simulink model "sampleModel152"  (Simulink 9.1)
settings: Solver=VariableStepAuto  StartTime=0.0  StopTime=10.0  RelTol=1e-3
undefined symbols (not defined in the file): DiscIntNeverNeededParam, Newton, Raphson
libraries: simulink x17
settings Model: Creator=DELL  LastModifiedBy=DELL
settings DataIOCC: SaveFormat=Dataset
settings OptimizationCC: LifeSpan=auto
settings DebuggingCC: UnderspecifiedInitializationDetection=Simplified  MergeDetectMultiDrivingBlocksExec=error  SFUnexpectedBacktrackingDiag=error  SFNoUnconditionalDefaultTransitionDiag=error  SFExecutionAtInitializationDiag=warning
settings HardwareCC: ProdBitPerPointer=64  ProdBitPerSizeT=64  ProdBitPerPtrDiffT=64  ProdLargestAtomicFloat=Float  ProdIntDivRoundTo=Zero  ProdEndianess=LittleEndian  ProdWordSize=64  ProdHWDeviceType=Intel->x86-64 (Windows64)
settings ModelReferenceCC: PropagateSignalLabelsOutOfModel=on
settings CodeAppCC: StateflowObjectComments=off
settings GRTTargetCC: TargetLangStandard=C99 (ISO)  CombineOutputUpdateFcns=on  GRTInterface=off
settings ConfigComp: CovMetricSettings=dwe  CovHtmlReporting=off  CovSaveCumulativeToWorkspaceVar=off  CovSaveSingleToWorkspaceVar=off  CovExternalEMLEnable=on

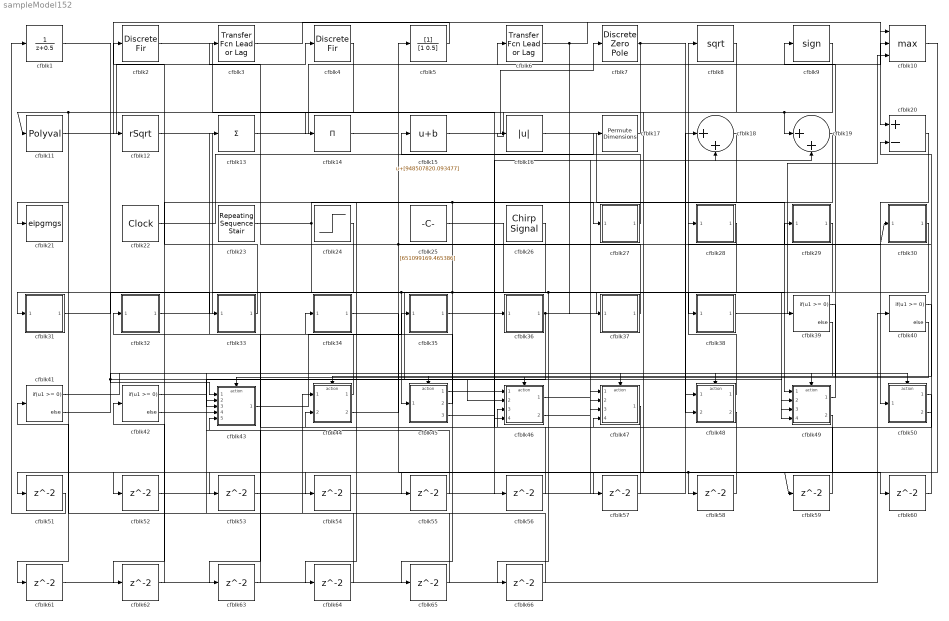
== system sampleModel152 ==
  cfblk1 : DiscreteTransferFcn  SampleTime=1
  cfblk10 : MinMax  Function=max  Inputs=3
  cfblk11 : Polyval  Coefs=[ +2.081618890e-019, -1.441693666e-014, +4.719686976e-010, -8.536869453e-006, +1.621573104e-001, -8.087801117e+001 ]
  cfblk12 : Sqrt  Operator=rSqrt  AlgorithmType=Newton-Raphson  SaturateOnIntegerOverflow=on
  cfblk13 : Sum  Inputs=+
  cfblk14 : Product  Inputs=*
  cfblk15 : Bias  Bias=[948507820.093477]
  cfblk16 : Abs
  cfblk17 : PermuteDimensions
  cfblk18 : Sum  Inputs=|++
  cfblk19 : Sum  Inputs=|++
  cfblk2 : DiscreteFir  SampleTime=1
  cfblk20 : Sum  Inputs=+-
  cfblk21 : ToWorkspace  VariableName=eipgmgs  SaveFormat=Timeseries  SampleTime=-1
  cfblk22 : DigitalClock
  cfblk23 : simulink/Sources/Repeating Sequence Stair  OutValues=[-106869927.062415, -61159748.069920]  tsamp=-1  OutMin=[]  OutMax=[]  OutDataTypeStr=double  OutputDataTypeScalingMode=double  OutDataType=fixdt(0,8)  ConRadixGroup=Best Precision: Vector-wise  OutScaling=2^-12
  cfblk24 : Step  Time=[15.000000]  Before=[-172570946.840389]  After=[-976275544.240260]  SampleTime=0
  cfblk25 : Constant  Value=[651099169.465386]  SampleTime=1
  cfblk26 : simulink/Sources/Chirp Signal  f1=[-435057966.777252]  T=[115531586.665615]  f2=[491750431.839140]
  cfblk27 : Subsystem
  cfblk28 : Subsystem
  cfblk29 : Subsystem
  cfblk3 : simulink/Discrete/Transfer Fcn Lead or Lag  PoleZ=0.95  ZeroZ=0.75  ICPrevOutput=0.0  ICPrevInput=0.0  DoSatur=off
      settings: SourceProductName=Simulink  SourceProductBaseCode=SL
  cfblk30 : Subsystem
  cfblk31 : Subsystem
  cfblk32 : Subsystem
  cfblk33 : Subsystem
  cfblk34 : Subsystem
  cfblk35 : Subsystem
  cfblk36 : Subsystem
  cfblk37 : Subsystem
  cfblk38 : Subsystem
  cfblk{39..42} (4 alike) : If  IfExpression=u1 >= 0  SampleTime=1
  cfblk4 : DiscreteFir  SampleTime=1
  cfblk43 : Subsystem  TreatAsAtomicUnit=on
  cfblk44 : Subsystem  TreatAsAtomicUnit=on
  cfblk45 : Subsystem  TreatAsAtomicUnit=on
  cfblk46 : Subsystem  TreatAsAtomicUnit=on
  cfblk47 : Subsystem  TreatAsAtomicUnit=on
  cfblk48 : Subsystem  TreatAsAtomicUnit=on
  cfblk49 : Subsystem  TreatAsAtomicUnit=on
  cfblk5 : DiscreteFilter  SampleTime=1
  cfblk50 : Subsystem  TreatAsAtomicUnit=on
  cfblk{51..66} (16 alike) : Delay  SampleTime=1
  cfblk6 : simulink/Discrete/Transfer Fcn Lead or Lag  PoleZ=0.95  ZeroZ=0.75  ICPrevOutput=0.0  ICPrevInput=0.0  DoSatur=off
      settings: SourceProductName=Simulink  SourceProductBaseCode=SL
  cfblk7 : DiscreteZeroPole  Poles=[0 0.5]  Gain=1
  cfblk8 : Sqrt  SaturateOnIntegerOverflow=on
  cfblk9 : Signum
  wires:
  cfblk13/1 -> cfblk6/1
  cfblk50/1(cfblk2) -> cfblk32/1(cfblk1)
  cfblk11/1 -> cfblk4/1
  cfblk27/1(cfblk2) -> cfblk15/1
  cfblk12/1 -> cfblk46/2(cfblk14)
  cfblk15/1 -> cfblk7/1
  cfblk6/1 -> cfblk20/1, cfblk37/1(cfblk1)
  cfblk5/1 -> cfblk12/1
  cfblk17/1 -> cfblk16/1
  cfblk33/1(cfblk2) -> cfblk2/1
  cfblk23/1 -> cfblk27/1(cfblk1), cfblk49/4(cfblk16)
  cfblk9/1 -> cfblk19/1, cfblk57/1
  cfblk1/1 -> cfblk48/2(cfblk8), cfblk43/1(cfblk1)
  cfblk8/1 -> cfblk11/1, cfblk21/1
  cfblk44/1(cfblk2) -> cfblk13/1
  cfblk22/1 -> cfblk5/1
  cfblk45/1(cfblk2) -> cfblk19/2
  cfblk48/1(cfblk2) -> cfblk8/1
  cfblk2/1 -> cfblk36/1(cfblk1)
  cfblk28/1(cfblk2) -> cfblk45/1(cfblk1), cfblk63/1
  cfblk43/1(cfblk2) -> cfblk35/1(cfblk1)
  cfblk3/1 -> cfblk10/1
  cfblk50/2(cfblk17) -> cfblk28/1(cfblk1)
  cfblk19/1 -> cfblk54/1, cfblk55/1
  cfblk16/1 -> cfblk49/1(cfblk1)
  cfblk14/1 -> cfblk10/2
  cfblk24/1 -> cfblk31/1(cfblk1)
  cfblk32/1(cfblk2) -> cfblk38/1(cfblk1)
  cfblk49/1(cfblk2) -> cfblk9/1
  cfblk7/1 -> cfblk49/2(cfblk14), cfblk14/1
  cfblk44/2(cfblk7) -> cfblk17/1, cfblk30/1(cfblk1)
  cfblk38/1(cfblk2) -> cfblk10/3
  cfblk31/1(cfblk2) -> cfblk33/1(cfblk1)
  cfblk36/1(cfblk2) -> cfblk39/1, cfblk43/3(cfblk11)
  cfblk20/1 -> cfblk50/1(cfblk1)
  cfblk30/1(cfblk2) -> cfblk64/1, cfblk65/1, cfblk66/1
  cfblk45/2(cfblk11) -> cfblk34/1(cfblk1)
  cfblk47/1(cfblk2) -> cfblk46/3(cfblk15)
  cfblk48/2(cfblk9) -> cfblk44/2(cfblk6)
  cfblk26/1 -> cfblk46/4(cfblk16)
  cfblk34/1(cfblk2) -> cfblk58/1, cfblk59/1
  cfblk46/1(cfblk2) -> cfblk29/1(cfblk1)
  cfblk37/1(cfblk2) -> cfblk3/1
  cfblk25/1 -> cfblk49/3(cfblk15)
  cfblk46/2(cfblk17) -> cfblk18/2
  cfblk39/1 -> cfblk43/Action
  cfblk39/2 -> cfblk44/Action
  cfblk40/1 -> cfblk45/Action
  cfblk40/2 -> cfblk46/Action
  cfblk41/1 -> cfblk47/Action
  cfblk41/2 -> cfblk48/Action
  cfblk42/1 -> cfblk49/Action
  cfblk42/2 -> cfblk50/Action
  cfblk4/1 -> cfblk51/1
  cfblk51/1 -> cfblk1/1
  cfblk10/1 -> cfblk52/1
  cfblk52/1 -> cfblk47/1(cfblk1)
  cfblk29/1(cfblk2) -> cfblk53/1
  cfblk53/1 -> cfblk48/1(cfblk1)
  cfblk54/1 -> cfblk18/1
  cfblk55/1 -> cfblk43/2(cfblk10)
  cfblk35/1(cfblk2) -> cfblk56/1
  cfblk56/1 -> cfblk46/1(cfblk1)
  cfblk57/1 -> cfblk47/3(cfblk14)
  cfblk58/1 -> cfblk47/2(cfblk13)
  cfblk59/1 -> cfblk47/4(cfblk15)
  cfblk45/3(cfblk12) -> cfblk60/1
  cfblk60/1 -> cfblk20/2
  cfblk49/2(cfblk17) -> cfblk61/1
  cfblk61/1 -> cfblk40/1
  cfblk18/1 -> cfblk62/1
  cfblk62/1 -> cfblk42/1
  cfblk63/1 -> cfblk43/5(cfblk13)
  cfblk64/1 -> cfblk44/1(cfblk1)
  cfblk65/1 -> cfblk41/1
  cfblk66/1 -> cfblk43/4(cfblk12)

== system sampleModel152/cfblk27 ==
  cfblk1 : Inport
  cfblk2 : Outport
  wires:
  cfblk1/1 -> cfblk2/1

== system sampleModel152/cfblk28 ==
  cfblk1 : Inport
  cfblk2 : Outport
  wires:
  cfblk1/1 -> cfblk2/1

== system sampleModel152/cfblk29 ==
  cfblk1 : Inport
  cfblk2 : Outport
  wires:
  cfblk1/1 -> cfblk2/1

== system sampleModel152/cfblk30 ==
  cfblk1 : Inport
  cfblk2 : Outport
  wires:
  cfblk1/1 -> cfblk2/1

== system sampleModel152/cfblk31 ==
  cfblk1 : Inport
  cfblk2 : Outport
  wires:
  cfblk1/1 -> cfblk2/1

== system sampleModel152/cfblk32 ==
  cfblk1 : Inport
  cfblk2 : Outport
  wires:
  cfblk1/1 -> cfblk2/1

== system sampleModel152/cfblk33 ==
  cfblk1 : Inport
  cfblk2 : Outport
  wires:
  cfblk1/1 -> cfblk2/1

== system sampleModel152/cfblk34 ==
  cfblk1 : Inport
  cfblk2 : Outport
  wires:
  cfblk1/1 -> cfblk2/1

== system sampleModel152/cfblk35 ==
  cfblk1 : Inport
  cfblk2 : Outport
  wires:
  cfblk1/1 -> cfblk2/1

== system sampleModel152/cfblk36 ==
  cfblk1 : Inport
  cfblk2 : Outport
  wires:
  cfblk1/1 -> cfblk2/1

== system sampleModel152/cfblk37 ==
  cfblk1 : Inport
  cfblk2 : Outport
  wires:
  cfblk1/1 -> cfblk2/1

== system sampleModel152/cfblk38 ==
  cfblk1 : Inport
  cfblk2 : Outport
  wires:
  cfblk1/1 -> cfblk2/1

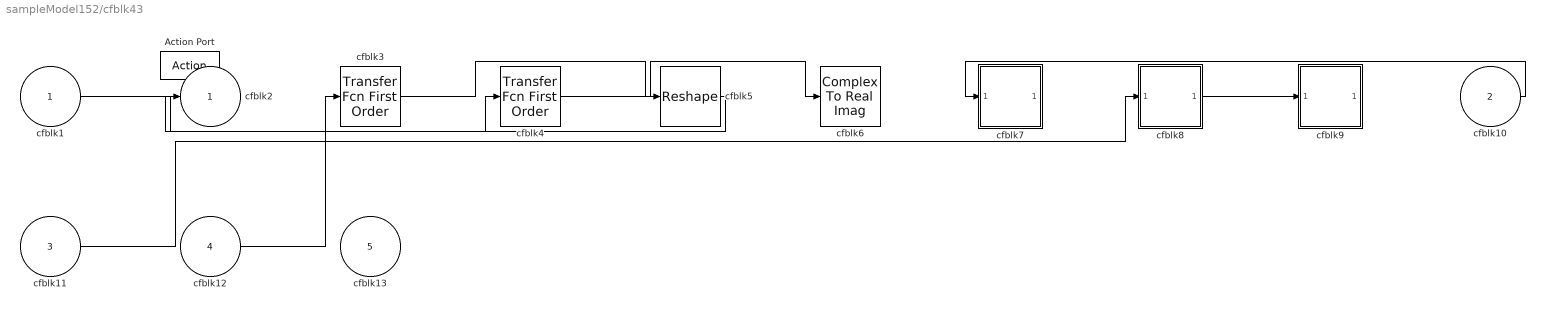
== system sampleModel152/cfblk43 ==
  cfblk1 : Inport
  cfblk10 : Inport  Port=2
  cfblk11 : Inport  Port=3
  cfblk12 : Inport  Port=4
  cfblk13 : Inport  Port=5
  Action Port : ActionPort  ActionType=then
  cfblk3 : simulink/Discrete/Transfer Fcn First Order  PoleZ=0.95  ICPrevOutput=0.0  DoSatur=off
      settings: SourceProductName=Simulink
  cfblk4 : simulink/Discrete/Transfer Fcn First Order  PoleZ=0.95  ICPrevOutput=0.0  DoSatur=off
      settings: SourceProductName=Simulink
  cfblk5 : Reshape
  cfblk6 : ComplexToRealImag
  cfblk7 : Subsystem
  cfblk8 : Subsystem
  cfblk9 : Subsystem
  cfblk2 : Outport
  wires:
  cfblk1/1 -> cfblk4/1
  cfblk11/1 -> cfblk8/1(cfblk1)
  cfblk4/1 -> cfblk6/1
  cfblk10/1 -> cfblk7/1(cfblk1)
  cfblk8/1(cfblk2) -> cfblk9/1(cfblk1)
  cfblk3/1 -> cfblk5/1
  cfblk12/1 -> cfblk3/1
  cfblk5/1 -> cfblk2/1

== system sampleModel152/cfblk44 ==
  cfblk1 : Inport
  cfblk6 : Inport  Port=2
  Action Port : ActionPort  ActionType=else
  cfblk3 : simulink/Continuous/PID Controller  Controller=PID  TimeDomain=Discrete-time  SampleTime=-1  IntegratorMethod=Forward Euler  FilterMethod=Forward Euler  Form=Parallel  UseFilter=on  ControllerParametersSource=internal  P=1  I=1  D=0  N=100  InitialConditionSource=internal  InitialConditionForIntegrator=0  InitialConditionForFilter=0  ExternalReset=none  LimitOutput=off  UpperSaturationLimit=inf  LowerSaturationLimit=-inf  LinearizeAsGain=off  AntiWindupMode=none  Kb=1  TrackingMode=off  Kt=1  PParamMin=[]  PParamMax=[]  IParamMin=[]  IParamMax=[]  DParamMin=[]  DParamMax=[]  NParamMin=[]  NParamMax=[]  KbParamMin=[]  KbParamMax=[]  KtParamMin=[]  KtParamMax=[]  POutMin=[]  POutMax=[]  IOutMin=[]  IOutMax=[]  DOutMin=[]  DOutMax=[]  NOutMin=[]  NOutMax=[]  KbOutMin=[]  KbOutMax=[]  KtOutMin=[]  KtOutMax=[]  IntegratorOutMin=[]  IntegratorOutMax=[]  FilterOutMin=[]  FilterOutMax=[]  SumOutMin=[]  SumOutMax=[]  SumI1OutMin=[]  SumI1OutMax=[]  SumI2OutMin=[]  SumI2OutMax=[]  SumI3OutMin=[]  SumI3OutMax=[]  SumDOutMin=[]  SumDOutMax=[]  SaturationOutMin=[]  SaturationOutMax=[]  IntegratorContinuousStateAttributes=''  IntegratorStateMustResolveToSignalObject=off  IntegratorRTWStateStorageClass=Auto  FilterContinuousStateAttributes=''  FilterStateMustResolveToSignalObject=off  FilterRTWStateStorageClass=Auto  DifferentiatorICPrevScaledInput=0  DifferentiatorOutMin=[]  DifferentiatorOutMax=[]  FilterDiffOutCoefMin=[]  FilterDiffOutCoefMax=[]  SumDenOutMin=[]  SumDenOutMax=[]  SumNumOutMin=[]  SumNumOutMax=[]  ReciprocalOutMin=[]  ReciprocalOutMax=[]  DivideOutMin=[]  DivideOutMax=[]  TunerSelectOption=Transfer Function Based (PID Tuner App)
  cfblk4 : DiscreteZeroPole  Poles=[0 0.5]  Gain=1  SampleTime=-1
  cfblk5 : simulink/Math Operations/Slider Gain  gain=1  low=0  high=2
  cfblk2 : Outport
  cfblk7 : Outport  Port=2
  wires:
  cfblk6/1 -> cfblk2/1
  cfblk5/1 -> cfblk7/1
  cfblk4/1 -> cfblk3/1
  cfblk1/1 -> cfblk4/1
  cfblk3/1 -> cfblk5/1

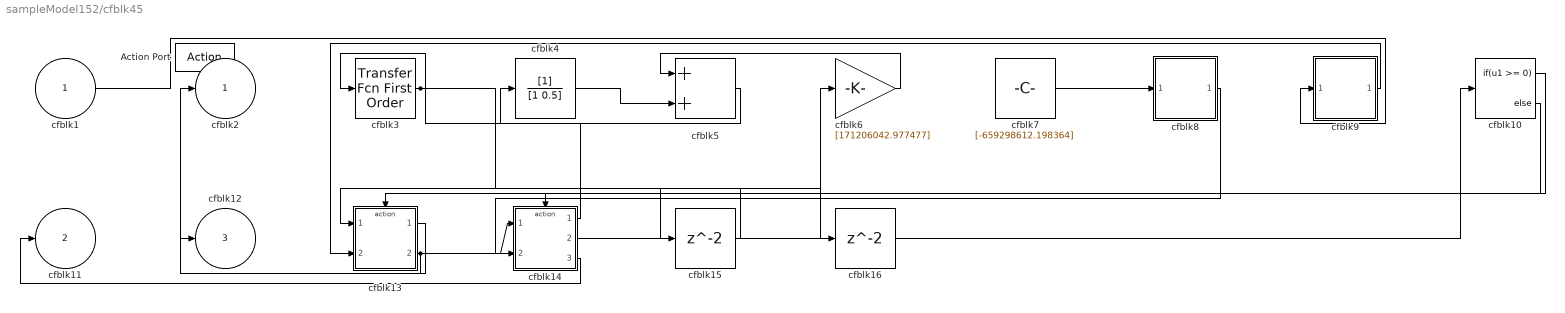
== system sampleModel152/cfblk45 ==
  cfblk1 : Inport
  Action Port : ActionPort  ActionType=then
  cfblk10 : If  IfExpression=u1 >= 0  SampleTime=1
  cfblk13 : Subsystem  TreatAsAtomicUnit=on
  cfblk14 : Subsystem  TreatAsAtomicUnit=on
  cfblk15 : Delay
  cfblk16 : Delay
  cfblk3 : simulink/Discrete/Transfer Fcn First Order  PoleZ=0.95  ICPrevOutput=0.0  DoSatur=off
      settings: SourceProductName=Simulink
  cfblk4 : DiscreteFilter
  cfblk5 : Sum
  cfblk6 : Gain  Gain=[171206042.977477]
  cfblk7 : Constant  Value=[-659298612.198364]  SampleTime=1
  cfblk8 : Subsystem
  cfblk9 : Subsystem
  cfblk2 : Outport
  cfblk11 : Outport  Port=2
  cfblk12 : Outport  Port=3
  wires:
  cfblk3/1 -> cfblk15/1, cfblk16/1
  cfblk6/1 -> cfblk5/1
  cfblk13/1(cfblk2) -> cfblk2/1
  cfblk5/1 -> cfblk3/1
  cfblk14/1(cfblk2) -> cfblk4/1
  cfblk14/2(cfblk8) -> cfblk6/1
  cfblk13/2(cfblk10) -> cfblk14/1(cfblk1), cfblk12/1
  cfblk9/1(cfblk2) -> cfblk13/2(cfblk9)
  cfblk1/1 -> cfblk9/1(cfblk1)
  cfblk14/3(cfblk9) -> cfblk11/1
  cfblk4/1 -> cfblk5/2
  cfblk8/1(cfblk2) -> cfblk14/2(cfblk7)
  cfblk7/1 -> cfblk8/1(cfblk1)
  cfblk10/1 -> cfblk13/Action
  cfblk10/2 -> cfblk14/Action
  cfblk15/1 -> cfblk13/1(cfblk1)
  cfblk16/1 -> cfblk10/1

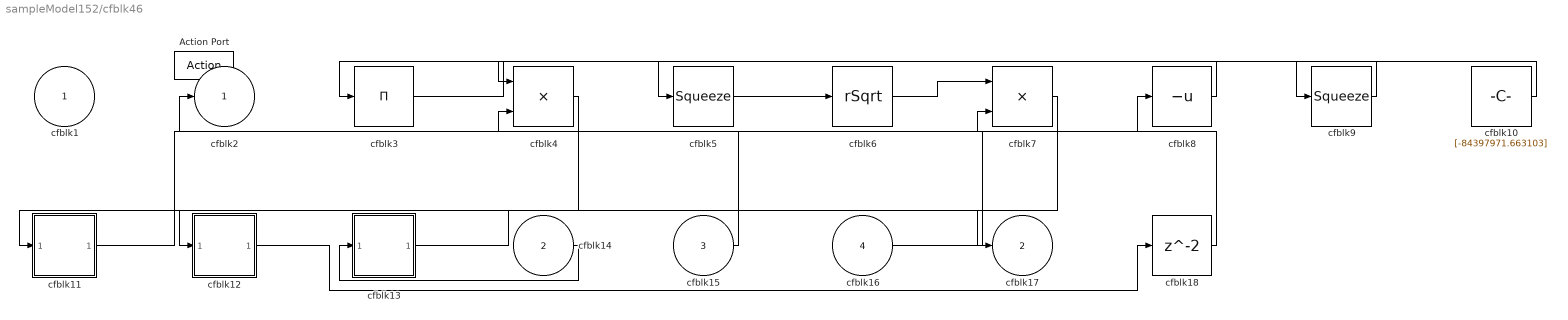
== system sampleModel152/cfblk46 ==
  cfblk1 : Inport
  cfblk14 : Inport  Port=2
  cfblk15 : Inport  Port=3
  cfblk16 : Inport  Port=4
  Action Port : ActionPort  ActionType=else
  cfblk10 : Constant  Value=[-84397971.663103]  SampleTime=1
  cfblk11 : Subsystem
  cfblk12 : Subsystem
  cfblk13 : Subsystem
  cfblk18 : Delay
  cfblk3 : Product  Inputs=*
  cfblk4 : Product
  cfblk5 : Squeeze
  cfblk6 : Sqrt  Operator=rSqrt  AlgorithmType=Newton-Raphson  SaturateOnIntegerOverflow=on
  cfblk7 : Product  Inputs=**
  cfblk8 : UnaryMinus
  cfblk9 : Squeeze
  cfblk2 : Outport
  cfblk17 : Outport  Port=2
  wires:
  cfblk4/1 -> cfblk11/1(cfblk1)
  cfblk14/1 -> cfblk13/1(cfblk1)
  cfblk16/1 -> cfblk8/1
  cfblk13/1(cfblk2) -> cfblk17/1
  cfblk15/1 -> cfblk2/1
  cfblk5/1 -> cfblk6/1
  cfblk10/1 -> cfblk5/1
  cfblk8/1 -> cfblk3/1
  cfblk7/1 -> cfblk12/1(cfblk1)
  cfblk6/1 -> cfblk7/1
  cfblk11/1(cfblk2) -> cfblk7/2
  cfblk3/1 -> cfblk9/1
  cfblk9/1 -> cfblk4/1
  cfblk12/1(cfblk2) -> cfblk18/1
  cfblk18/1 -> cfblk4/2

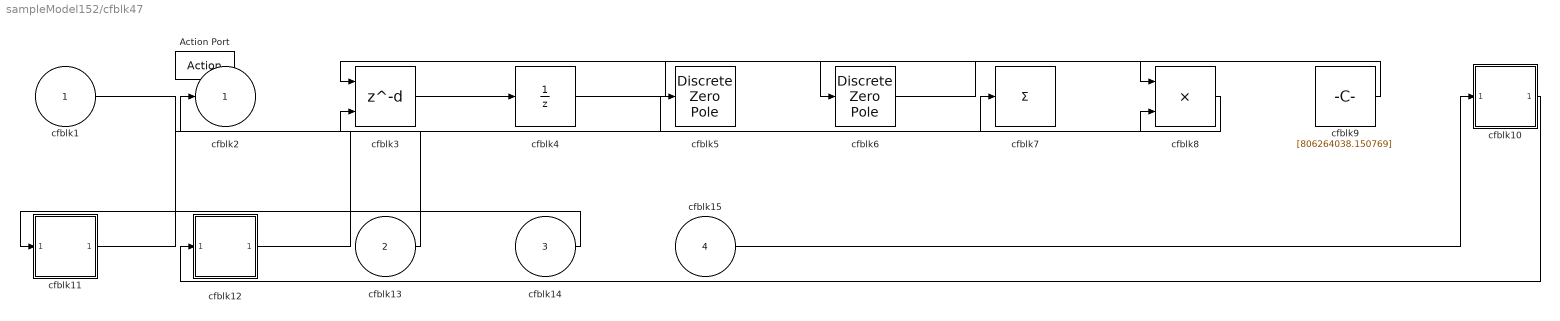
== system sampleModel152/cfblk47 ==
  cfblk1 : Inport
  cfblk13 : Inport  Port=2
  cfblk14 : Inport  Port=3
  cfblk15 : Inport  Port=4
  Action Port : ActionPort  ActionType=then
  cfblk10 : Subsystem
  cfblk11 : Subsystem
  cfblk12 : Subsystem
  cfblk3 : Delay  DelayLengthSource=Input port
      settings: InputPortMap=u0,p1
  cfblk4 : UnitDelay  SampleTime=-1
  cfblk5 : DiscreteZeroPole  Poles=[0 0.5]  Gain=1  SampleTime=-1
  cfblk6 : DiscreteZeroPole  Poles=[0 0.5]  Gain=1  SampleTime=-1
  cfblk7 : Sum  Inputs=+
  cfblk8 : Product
  cfblk9 : Constant  Value=[806264038.150769]  SampleTime=1
  cfblk2 : Outport
  wires:
  cfblk12/1(cfblk2) -> cfblk7/1
  cfblk9/1 -> cfblk3/1
  cfblk15/1 -> cfblk10/1(cfblk1)
  cfblk10/1(cfblk2) -> cfblk12/1(cfblk1)
  cfblk6/1 -> cfblk8/1
  cfblk3/1 -> cfblk4/1
  cfblk11/1(cfblk2) -> cfblk8/2
  cfblk8/1 -> cfblk2/1
  cfblk14/1 -> cfblk11/1(cfblk1)
  cfblk4/1 -> cfblk6/1
  cfblk1/1 -> cfblk5/1
  cfblk13/1 -> cfblk3/2

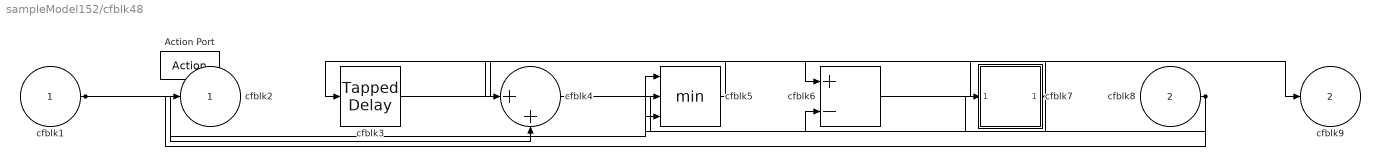
== system sampleModel152/cfblk48 ==
  cfblk1 : Inport
  cfblk8 : Inport  Port=2
  Action Port : ActionPort  ActionType=else
  cfblk3 : simulink/Discrete/Tapped Delay  vinit=0.0  samptime=-1  NumDelays=1  DelayOrder=Oldest  includeCurrent=off
  cfblk4 : Sum  Inputs=|++
  cfblk5 : MinMax  Inputs=3
  cfblk6 : Sum  Inputs=+-
  cfblk7 : Subsystem
  cfblk2 : Outport
  cfblk9 : Outport  Port=2
  wires:
  cfblk6/1 -> cfblk9/1
  cfblk5/1 -> cfblk3/1
  cfblk8/1 -> cfblk7/1(cfblk1), cfblk5/3, cfblk2/1
  cfblk1/1 -> cfblk5/1, cfblk4/2
  cfblk3/1 -> cfblk6/1
  cfblk7/1(cfblk2) -> cfblk4/1, cfblk5/2
  cfblk4/1 -> cfblk6/2

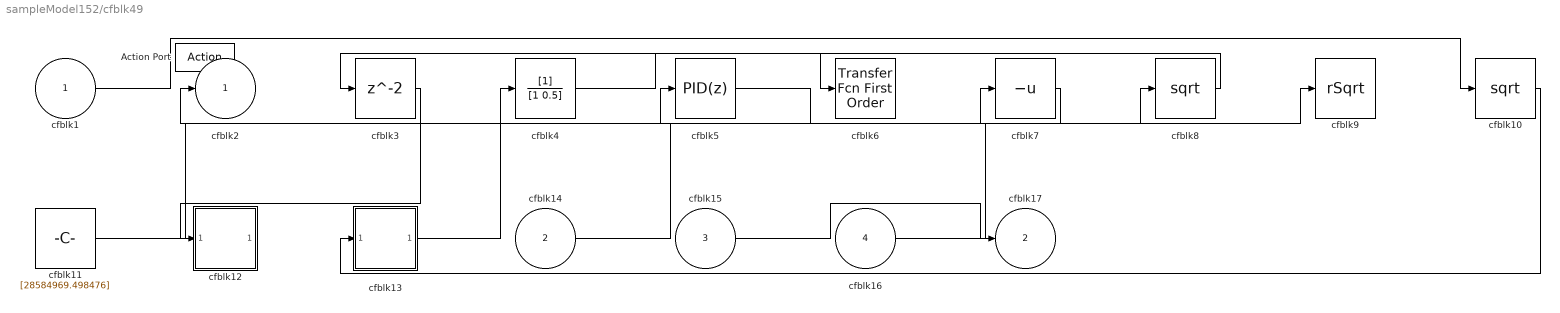
== system sampleModel152/cfblk49 ==
  cfblk1 : Inport
  cfblk14 : Inport  Port=2
  cfblk15 : Inport  Port=3
  cfblk16 : Inport  Port=4
  Action Port : ActionPort  ActionType=then
  cfblk10 : Sqrt  SaturateOnIntegerOverflow=on
  cfblk11 : Constant  Value=[28584969.498476]  SampleTime=1
  cfblk12 : Subsystem
  cfblk13 : Subsystem
  cfblk3 : Delay
  cfblk4 : DiscreteFilter
  cfblk5 : simulink/Continuous/PID Controller  Controller=PID  TimeDomain=Discrete-time  SampleTime=-1  IntegratorMethod=Forward Euler  FilterMethod=Forward Euler  Form=Parallel  UseFilter=on  ControllerParametersSource=internal  P=1  I=1  D=0  N=100  InitialConditionSource=internal  InitialConditionForIntegrator=0  InitialConditionForFilter=0  ExternalReset=none  LimitOutput=off  UpperSaturationLimit=inf  LowerSaturationLimit=-inf  LinearizeAsGain=off  AntiWindupMode=none  Kb=1  TrackingMode=off  Kt=1  PParamMin=[]  PParamMax=[]  IParamMin=[]  IParamMax=[]  DParamMin=[]  DParamMax=[]  NParamMin=[]  NParamMax=[]  KbParamMin=[]  KbParamMax=[]  KtParamMin=[]  KtParamMax=[]  POutMin=[]  POutMax=[]  IOutMin=[]  IOutMax=[]  DOutMin=[]  DOutMax=[]  NOutMin=[]  NOutMax=[]  KbOutMin=[]  KbOutMax=[]  KtOutMin=[]  KtOutMax=[]  IntegratorOutMin=[]  IntegratorOutMax=[]  FilterOutMin=[]  FilterOutMax=[]  SumOutMin=[]  SumOutMax=[]  SumI1OutMin=[]  SumI1OutMax=[]  SumI2OutMin=[]  SumI2OutMax=[]  SumI3OutMin=[]  SumI3OutMax=[]  SumDOutMin=[]  SumDOutMax=[]  SaturationOutMin=[]  SaturationOutMax=[]  IntegratorContinuousStateAttributes=''  IntegratorStateMustResolveToSignalObject=off  IntegratorRTWStateStorageClass=Auto  FilterContinuousStateAttributes=''  FilterStateMustResolveToSignalObject=off  FilterRTWStateStorageClass=Auto  DifferentiatorICPrevScaledInput=0  DifferentiatorOutMin=[]  DifferentiatorOutMax=[]  FilterDiffOutCoefMin=[]  FilterDiffOutCoefMax=[]  SumDenOutMin=[]  SumDenOutMax=[]  SumNumOutMin=[]  SumNumOutMax=[]  ReciprocalOutMin=[]  ReciprocalOutMax=[]  DivideOutMin=[]  DivideOutMax=[]  TunerSelectOption=Transfer Function Based (PID Tuner App)
  cfblk6 : simulink/Discrete/Transfer Fcn First Order  PoleZ=0.95  ICPrevOutput=0.0  DoSatur=off
      settings: SourceProductName=Simulink
  cfblk7 : UnaryMinus
  cfblk8 : Sqrt  SaturateOnIntegerOverflow=on
  cfblk9 : Sqrt  Operator=rSqrt  AlgorithmType=Newton-Raphson  SaturateOnIntegerOverflow=on
  cfblk2 : Outport
  cfblk17 : Outport  Port=2
  wires:
  cfblk8/1 -> cfblk3/1
  cfblk11/1 -> cfblk5/1
  cfblk4/1 -> cfblk6/1
  cfblk5/1 -> cfblk9/1
  cfblk1/1 -> cfblk10/1
  cfblk16/1 -> cfblk8/1
  cfblk10/1 -> cfblk13/1(cfblk1)
  cfblk7/1 -> cfblk2/1
  cfblk13/1(cfblk2) -> cfblk4/1
  cfblk3/1 -> cfblk12/1(cfblk1)
  cfblk14/1 -> cfblk7/1
  cfblk15/1 -> cfblk17/1

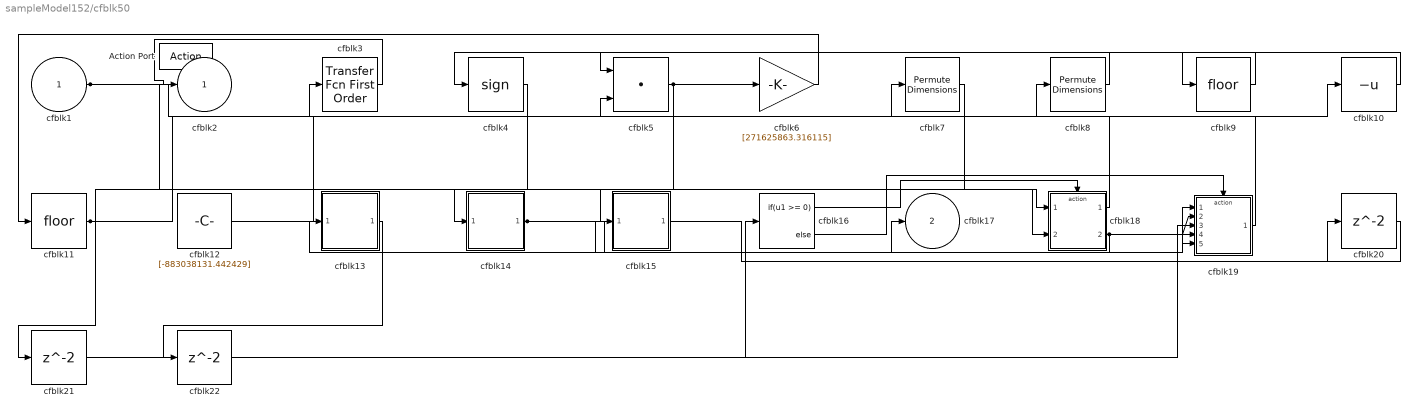
== system sampleModel152/cfblk50 ==
  cfblk1 : Inport
  Action Port : ActionPort  ActionType=else
  cfblk10 : UnaryMinus
  cfblk11 : Rounding
  cfblk12 : Constant  Value=[-883038131.442429]  SampleTime=1
  cfblk13 : Subsystem
  cfblk14 : Subsystem
  cfblk15 : Subsystem
  cfblk16 : If  IfExpression=u1 >= 0  SampleTime=1
  cfblk18 : Subsystem  TreatAsAtomicUnit=on
  cfblk19 : Subsystem  TreatAsAtomicUnit=on
  cfblk20 : Delay
  cfblk21 : Delay
  cfblk22 : Delay
  cfblk3 : simulink/Discrete/Transfer Fcn First Order  PoleZ=0.95  ICPrevOutput=0.0  DoSatur=off
      settings: SourceProductName=Simulink
  cfblk4 : Signum
  cfblk5 : DotProduct  InputSameDT=on  OutDataTypeStr=Inherit: Inherit via internal rule
  cfblk6 : Gain  Gain=[271625863.316115]
  cfblk7 : PermuteDimensions
  cfblk8 : PermuteDimensions
  cfblk9 : Rounding
  cfblk2 : Outport
  cfblk17 : Outport  Port=2
  wires:
  cfblk1/1 -> cfblk10/1, cfblk18/2(cfblk11)
  cfblk3/1 -> cfblk2/1
  cfblk6/1 -> cfblk11/1
  cfblk18/1(cfblk2) -> cfblk7/1
  cfblk9/1 -> cfblk5/1
  cfblk14/1(cfblk2) -> cfblk19/1(cfblk1), cfblk19/5(cfblk8)
  cfblk10/1 -> cfblk9/1
  cfblk11/1 -> cfblk18/1(cfblk1), cfblk3/1
  cfblk18/2(cfblk12) -> cfblk19/2(cfblk5), cfblk13/1(cfblk1), cfblk17/1
  cfblk8/1 -> cfblk4/1
  cfblk5/1 -> cfblk6/1, cfblk14/1(cfblk1)
  cfblk7/1 -> cfblk15/1(cfblk1)
  cfblk19/1(cfblk2) -> cfblk8/1
  cfblk12/1 -> cfblk5/2
  cfblk16/1 -> cfblk18/Action
  cfblk16/2 -> cfblk19/Action
  cfblk15/1(cfblk2) -> cfblk20/1
  cfblk20/1 -> cfblk19/3(cfblk6)
  cfblk4/1 -> cfblk21/1
  cfblk21/1 -> cfblk16/1
  cfblk13/1(cfblk2) -> cfblk22/1
  cfblk22/1 -> cfblk19/4(cfblk7)

== system sampleModel152/cfblk43/cfblk7 ==
  cfblk1 : Inport
  cfblk2 : Outport
  wires:
  cfblk1/1 -> cfblk2/1

== system sampleModel152/cfblk43/cfblk8 ==
  cfblk1 : Inport
  cfblk2 : Outport
  wires:
  cfblk1/1 -> cfblk2/1

== system sampleModel152/cfblk43/cfblk9 ==
  cfblk1 : Inport
  cfblk2 : Outport
  wires:
  cfblk1/1 -> cfblk2/1

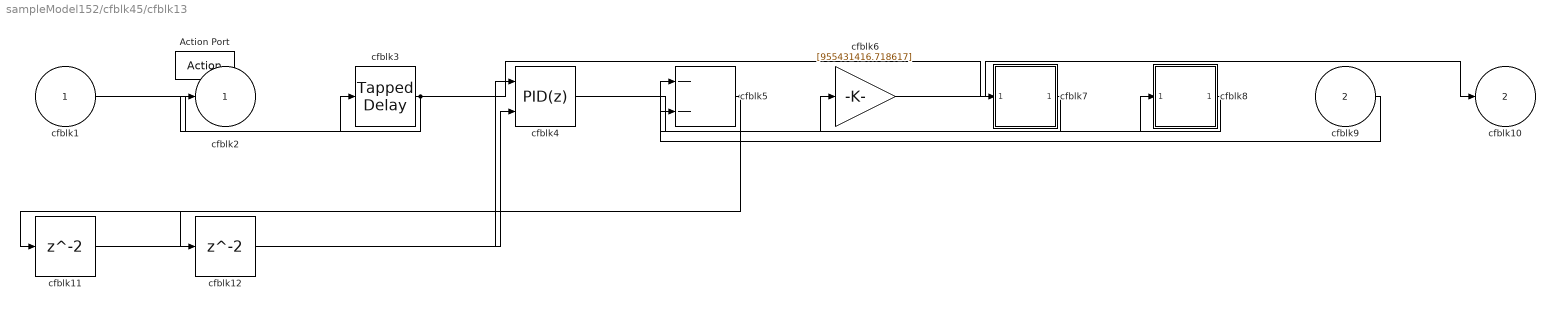
== system sampleModel152/cfblk45/cfblk13 ==
  cfblk1 : Inport
  cfblk9 : Inport  Port=2
  Action Port : ActionPort  ActionType=then
  cfblk11 : Delay
  cfblk12 : Delay
  cfblk3 : simulink/Discrete/Tapped Delay  vinit=0.0  samptime=-1  NumDelays=1  DelayOrder=Oldest  includeCurrent=off
  cfblk4 : simulink/Continuous/PID Controller (2DOF)  Controller=PID  TimeDomain=Discrete-time  SampleTime=-1  IntegratorMethod=Forward Euler  FilterMethod=Forward Euler  Form=Parallel  UseFilter=on  ControllerParametersSource=internal  P=1  I=1  D=0  N=100  b=1  c=1  InitialConditionSource=internal  InitialConditionForIntegrator=0  InitialConditionForFilter=0  ExternalReset=none  LimitOutput=off  UpperSaturationLimit=inf  LowerSaturationLimit=-inf  LinearizeAsGain=off  AntiWindupMode=none  Kb=1  TrackingMode=off  Kt=1  PParamMin=[]  PParamMax=[]  IParamMin=[]  IParamMax=[]  DParamMin=[]  DParamMax=[]  NParamMin=[]  NParamMax=[]  bParamMin=[]  bParamMax=[]  cParamMin=[]  cParamMax=[]  KbParamMin=[]  KbParamMax=[]  KtParamMin=[]  KtParamMax=[]  POutMin=[]  POutMax=[]  IOutMin=[]  IOutMax=[]  DOutMin=[]  DOutMax=[]  NOutMin=[]  NOutMax=[]  bOutMin=[]  bOutMax=[]  cOutMin=[]  cOutMax=[]  KbOutMin=[]  KbOutMax=[]  KtOutMin=[]  KtOutMax=[]  IntegratorOutMin=[]  IntegratorOutMax=[]  FilterOutMin=[]  FilterOutMax=[]  SumOutMin=[]  SumOutMax=[]  Sum1OutMin=[]  Sum1OutMax=[]  Sum2OutMin=[]  Sum2OutMax=[]  Sum3OutMin=[]  Sum3OutMax=[]  SumI1OutMin=[]  SumI1OutMax=[]  SumI2OutMin=[]  SumI2OutMax=[]  SumI3OutMin=[]  SumI3OutMax=[]  SumDOutMin=[]  SumDOutMax=[]  SaturationOutMin=[]  SaturationOutMax=[]  IntegratorContinuousStateAttributes=''  IntegratorStateMustResolveToSignalObject=off  IntegratorRTWStateStorageClass=Auto  FilterContinuousStateAttributes=''  FilterStateMustResolveToSignalObject=off  FilterRTWStateStorageClass=Auto  DifferentiatorICPrevScaledInput=0  DifferentiatorOutMin=[]  DifferentiatorOutMax=[]  FilterDiffOutCoefMin=[]  FilterDiffOutCoefMax=[]  SumDenOutMin=[]  SumDenOutMax=[]  SumNumOutMin=[]  SumNumOutMax=[]  ReciprocalOutMin=[]  ReciprocalOutMax=[]  DivideOutMin=[]  DivideOutMax=[]  TunerSelectOption=Transfer Function Based (PID Tuner App)
  cfblk5 : Sum  Inputs=--
  cfblk6 : Gain  Gain=[955431416.718617]
  cfblk7 : Subsystem
  cfblk8 : Subsystem
  cfblk2 : Outport
  cfblk10 : Outport  Port=2
  wires:
  cfblk6/1 -> cfblk10/1
  cfblk7/1(cfblk2) -> cfblk6/1
  cfblk9/1 -> cfblk5/1
  cfblk1/1 -> cfblk3/1
  cfblk3/1 -> cfblk7/1(cfblk1), cfblk2/1
  cfblk4/1 -> cfblk8/1(cfblk1)
  cfblk8/1(cfblk2) -> cfblk5/2
  cfblk5/1 -> cfblk11/1, cfblk12/1
  cfblk11/1 -> cfblk4/1
  cfblk12/1 -> cfblk4/2

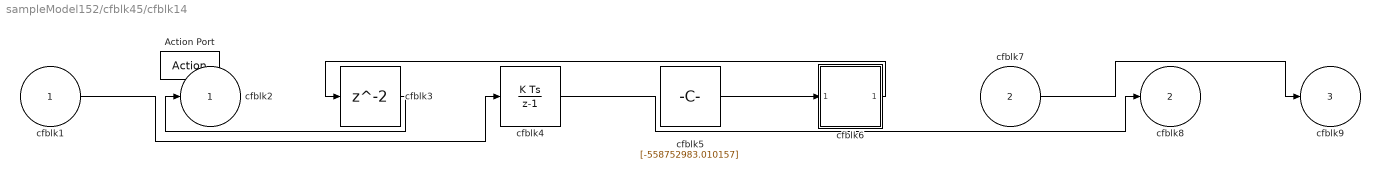
== system sampleModel152/cfblk45/cfblk14 ==
  cfblk1 : Inport
  cfblk7 : Inport  Port=2
  Action Port : ActionPort  ActionType=else
  cfblk3 : Delay
  cfblk4 : DiscreteIntegrator  SampleTime=-1  ICPrevOutput=DiscIntNeverNeededParam  ICPrevScaledInput=DiscIntNeverNeededParam
  cfblk5 : Constant  Value=[-558752983.010157]  SampleTime=1
  cfblk6 : Subsystem
  cfblk2 : Outport
  cfblk8 : Outport  Port=2
  cfblk9 : Outport  Port=3
  wires:
  cfblk6/1(cfblk2) -> cfblk3/1
  cfblk4/1 -> cfblk8/1
  cfblk5/1 -> cfblk6/1(cfblk1)
  cfblk7/1 -> cfblk9/1
  cfblk3/1 -> cfblk2/1
  cfblk1/1 -> cfblk4/1

== system sampleModel152/cfblk45/cfblk8 ==
  cfblk1 : Inport
  cfblk2 : Outport
  wires:
  cfblk1/1 -> cfblk2/1

== system sampleModel152/cfblk45/cfblk9 ==
  cfblk1 : Inport
  cfblk2 : Outport
  wires:
  cfblk1/1 -> cfblk2/1

== system sampleModel152/cfblk46/cfblk11 ==
  cfblk1 : Inport
  cfblk2 : Outport
  wires:
  cfblk1/1 -> cfblk2/1

== system sampleModel152/cfblk46/cfblk12 ==
  cfblk1 : Inport
  cfblk2 : Outport
  wires:
  cfblk1/1 -> cfblk2/1

== system sampleModel152/cfblk46/cfblk13 ==
  cfblk1 : Inport
  cfblk2 : Outport
  wires:
  cfblk1/1 -> cfblk2/1

== system sampleModel152/cfblk47/cfblk10 ==
  cfblk1 : Inport
  cfblk2 : Outport
  wires:
  cfblk1/1 -> cfblk2/1

== system sampleModel152/cfblk47/cfblk11 ==
  cfblk1 : Inport
  cfblk2 : Outport
  wires:
  cfblk1/1 -> cfblk2/1

== system sampleModel152/cfblk47/cfblk12 ==
  cfblk1 : Inport
  cfblk2 : Outport
  wires:
  cfblk1/1 -> cfblk2/1

== system sampleModel152/cfblk48/cfblk7 ==
  cfblk1 : Inport
  cfblk2 : Outport
  wires:
  cfblk1/1 -> cfblk2/1

== system sampleModel152/cfblk49/cfblk12 ==
  cfblk1 : Inport
  cfblk2 : Outport
  wires:
  cfblk1/1 -> cfblk2/1

== system sampleModel152/cfblk49/cfblk13 ==
  cfblk1 : Inport
  cfblk2 : Outport
  wires:
  cfblk1/1 -> cfblk2/1

== system sampleModel152/cfblk50/cfblk13 ==
  cfblk1 : Inport
  cfblk2 : Outport
  wires:
  cfblk1/1 -> cfblk2/1

== system sampleModel152/cfblk50/cfblk14 ==
  cfblk1 : Inport
  cfblk2 : Outport
  wires:
  cfblk1/1 -> cfblk2/1

== system sampleModel152/cfblk50/cfblk15 ==
  cfblk1 : Inport
  cfblk2 : Outport
  wires:
  cfblk1/1 -> cfblk2/1

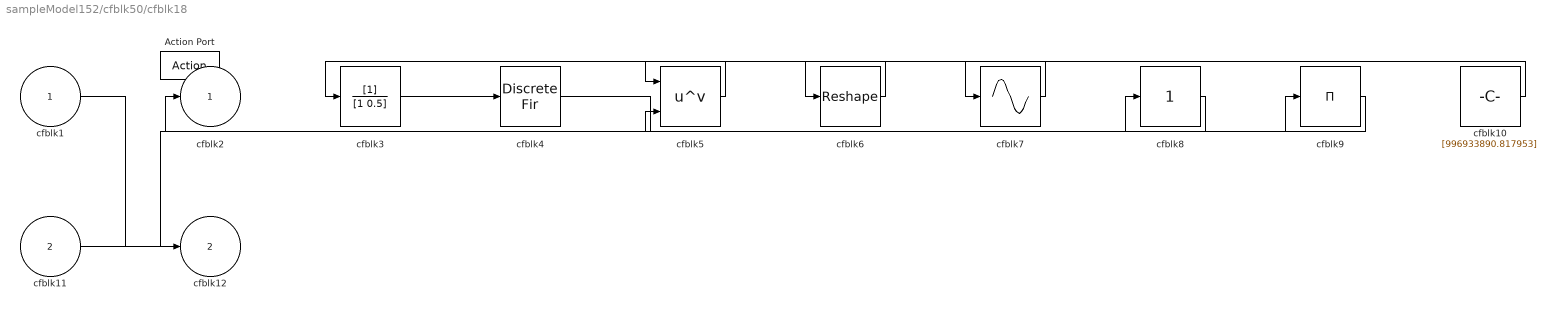
== system sampleModel152/cfblk50/cfblk18 ==
  cfblk1 : Inport
  cfblk11 : Inport  Port=2
  Action Port : ActionPort  ActionType=then
  cfblk10 : Constant  Value=[996933890.817953]  SampleTime=1
  cfblk3 : DiscreteFilter
  cfblk4 : DiscreteFir
  cfblk5 : Math  Operator=pow  SaturateOnIntegerOverflow=on
  cfblk6 : Reshape
  cfblk7 : Sin  TimeSource=Use external signal  SampleTime=0
  cfblk8 : simulink/Math Operations/Slider Gain  gain=1  low=0  high=2
  cfblk9 : Product  Inputs=*
  cfblk2 : Outport
  cfblk12 : Outport  Port=2
  wires:
  cfblk7/1 -> cfblk6/1
  cfblk4/1 -> cfblk9/1
  cfblk1/1 -> cfblk12/1
  cfblk6/1 -> cfblk5/1
  cfblk8/1 -> cfblk5/2
  cfblk3/1 -> cfblk4/1
  cfblk10/1 -> cfblk7/1
  cfblk5/1 -> cfblk3/1
  cfblk11/1 -> cfblk8/1
  cfblk9/1 -> cfblk2/1

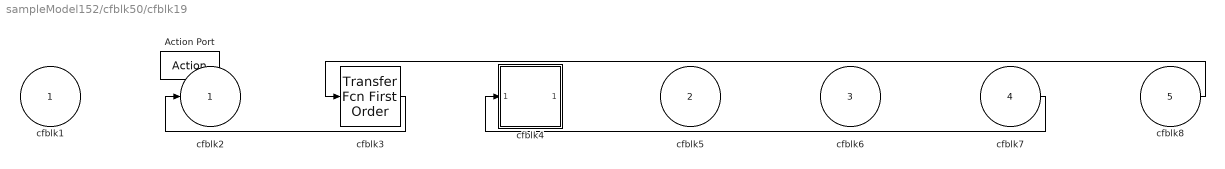
== system sampleModel152/cfblk50/cfblk19 ==
  cfblk1 : Inport
  cfblk5 : Inport  Port=2
  cfblk6 : Inport  Port=3
  cfblk7 : Inport  Port=4
  cfblk8 : Inport  Port=5
  Action Port : ActionPort  ActionType=else
  cfblk3 : simulink/Discrete/Transfer Fcn First Order  PoleZ=0.95  ICPrevOutput=0.0  DoSatur=off
      settings: SourceProductName=Simulink
  cfblk4 : Subsystem
  cfblk2 : Outport
  wires:
  cfblk3/1 -> cfblk2/1
  cfblk8/1 -> cfblk3/1
  cfblk7/1 -> cfblk4/1(cfblk1)

== system sampleModel152/cfblk45/cfblk13/cfblk7 ==
  cfblk1 : Inport
  cfblk2 : Outport
  wires:
  cfblk1/1 -> cfblk2/1

== system sampleModel152/cfblk45/cfblk13/cfblk8 ==
  cfblk1 : Inport
  cfblk2 : Outport
  wires:
  cfblk1/1 -> cfblk2/1

== system sampleModel152/cfblk45/cfblk14/cfblk6 ==
  cfblk1 : Inport
  cfblk2 : Outport
  wires:
  cfblk1/1 -> cfblk2/1

== system sampleModel152/cfblk50/cfblk19/cfblk4 ==
  cfblk1 : Inport
  cfblk2 : Outport
  wires:
  cfblk1/1 -> cfblk2/1
